simulink model "V2GStronge2_published_controller"  (R2024a)
settings: Solver=odeN  StartTime=0.0  StopTime=36000  FixedStep=10
model workspace (MAT data in the model file):
  Soc = 75
undefined symbols (not defined in the file): Ion, Lithium
libraries: spsMosfetLib x14, spsSeriesRLCBranchLib x14, slpidlib x8, spsBatteryLib x4, spsPWMGeneratorDCDCLib x4, spsCurrentMeasurementLib x3, spsAlphaBetaZerotodq0Lib x2, spsGroundLib x1, spsPWMGenerator2LevelLib x1, eePowerMeasurement x1, spsThreePhaseVIMeasurementLib x1, spsThreePhaseSourceLib x1
(part 2 of 2)

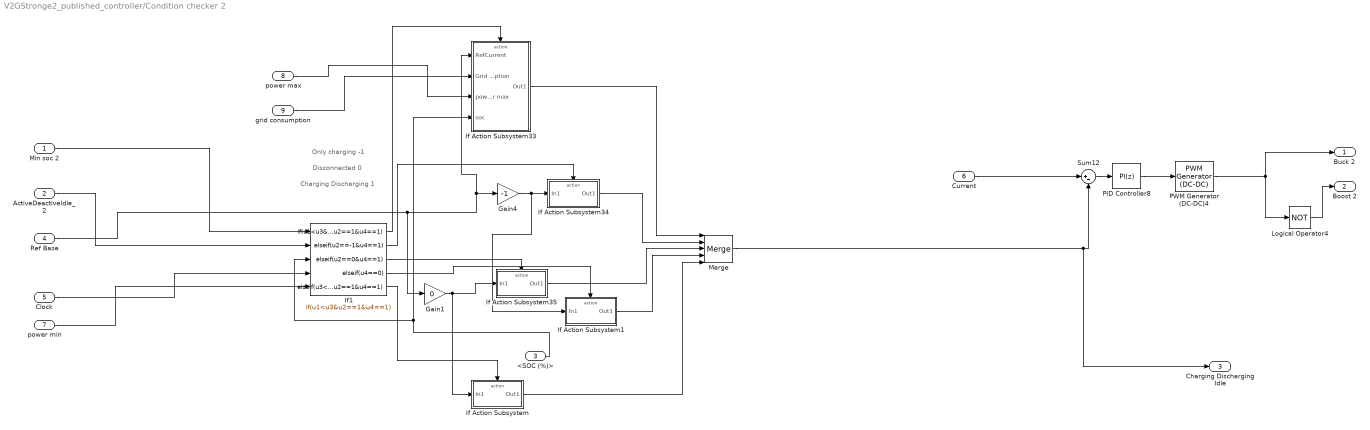
== system V2GStronge2_published_controller/Condition checker 2 ==
  note: Charging Discharging 1
  note: Disconnected 0
  note: Only charging -1
  Min soc 2 : Inport
  ActiveDeactiveIdle_2 : Inport  Port=2
  <SOC (%)> : Inport  Port=3
  Ref Base : Inport  Port=4
  Clock : Inport  Port=5
  Current : Inport  Port=6
  power min : Inport  Port=7
  power max : Inport  Port=8
  grid consumption : Inport  Port=9
  Gain1 : Gain  Gain=0
  Gain4 : Gain  Gain=-1
  If Action Subsystem : Subsystem  TreatAsAtomicUnit=on
  If Action Subsystem1 : Subsystem  TreatAsAtomicUnit=on
  If Action Subsystem33 : Subsystem  TreatAsAtomicUnit=on
  If Action Subsystem34 : Subsystem  TreatAsAtomicUnit=on
  If Action Subsystem35 : Subsystem  TreatAsAtomicUnit=on
  If1 : If  NumInputs=5  IfExpression=u1<u3&u2==1&u4==1  ElseIfExpressions=u2==-1&u4==1,u2==0&u4==1,u4==0,u3<u1&u2==1&u4==1  ShowElse=off
  Logical Operator4 : Logic  Operator=NOT  AllPortsSameDT=off  OutDataTypeStr=boolean
  Merge : Merge  Inputs=5
  PID Controller8 : slpidlib/PID Controller  Controller=PI  Form=Parallel  TimeDomain=Discrete-time  UseExternalTs=off  SampleTime=-1  IntegratorMethod=Forward Euler  FilterMethod=Forward Euler  ControllerParametersSource=internal  P=0.005  I=10  UseKiTs=off  D=0  UseExternalDerivativeSource=off  N=100  UseFilter=on  TunerSelectOption=Transfer Function Based (PID Tuner App)  InitialConditionSource=internal  InitialConditionForIntegrator=0  InitialConditionForFilter=0  DifferentiatorICPrevScaledInput=0  ExternalReset=none  TrackingMode=off  Kt=1  LimitOutput=on  SatLimitsSource=internal  UpperSaturationLimit=0.95  LowerSaturationLimit=0  LinearizeAsGain=on  AntiWindupMode=none  Kb=1  LimitIntegrator=off  UpperIntegratorSaturationLimit=inf  LowerIntegratorSaturationLimit=-inf  POutMin=[]  POutMax=[]  IOutMin=[]  IOutMax=[]  DOutMin=[]  DOutMax=[]  NOutMin=[]  NOutMax=[]  SumOutMin=[]  SumOutMax=[]  SaturationOutMin=[]  SaturationOutMax=[]  PParamMin=[]  PParamMax=[]  IParamMin=[]  IParamMax=[]  DParamMin=[]  DParamMax=[]  NParamMin=[]  NParamMax=[]  KbParamMin=[]  KbParamMax=[]  KtParamMin=[]  KtParamMax=[]  KbOutMin=[]  KbOutMax=[]  KtOutMin=[]  KtOutMax=[]  IntegratorOutMin=[]  IntegratorOutMax=[]  FilterOutMin=[]  FilterOutMax=[]  SumI1OutMin=[]  SumI1OutMax=[]  SumI2OutMin=[]  SumI2OutMax=[]  SumI3OutMin=[]  SumI3OutMax=[]  SumI4OutMin=[]  SumI4OutMax=[]  SumDOutMin=[]  SumDOutMax=[]  DifferentiatorOutMin=[]  DifferentiatorOutMax=[]  FilterDiffOutCoefMin=[]  FilterDiffOutCoefMax=[]  ReciprocalOutMin=[]  ReciprocalOutMax=[]  SumDenOutMin=[]  SumDenOutMax=[]  SumNumOutMin=[]  SumNumOutMax=[]  DivideOutMin=[]  DivideOutMax=[]  UdiffTsProdOutMin=[]  UdiffTsProdOutMax=[]  NTsProdOutMin=[]  NTsProdOutMax=[]  UintegralTsProdOutMin=[]  UintegralTsProdOutMax=[]  UngainTsProdOutMin=[]  UngainTsProdOutMax=[]  ClampingZeroOutDataTypeStr=Inherit: Inherit via back propagation  ClampingZeroOutMin=[]  ClampingZeroOutMax=[]  FilterDenConstantOutDataTypeStr=Inherit: Inherit via back propagation  FilterDenConstantOutMin=[]  FilterDenConstantOutMax=[]  PCopyOutDataTypeStr=Inherit: Inherit via back propagation  PCopyOutMin=[]  PCopyOutMax=[]  NCopyOutDataTypeStr=Inherit: Inherit via back propagation  NCopyOutMin=[]  NCopyOutMax=[]  IntegratorContinuousStateAttributes=''  IntegratorStateMustResolveToSignalObject=off  IntegratorRTWStateStorageClass=Auto  FilterContinuousStateAttributes=''  FilterStateMustResolveToSignalObject=off  FilterRTWStateStorageClass=Auto  ParallelPVariant=InternalParameters  IdealPVariant=Disabled  IVariant=InternalParameters  DVariant=Disabled  IntegratorVariant=Discrete  SatVariant=Enabled  AWVariant=Passthrough  PCopyVariant=Disabled  TRVariant=Disabled  FdbkBlocksVariant=Forward  IdealPFdbkVariant=Disabled  SatFdbkVariant=Disabled  DerivativeFilterVariant=Disabled  NVariant=Disabled  NCopyVariant=Disabled_SignalSpec  FilterICVariant=Disabled  IntegratorICVariant=InternalICs  ExternalResetVariant=Disabled  TRSumVariant=Passthrough  SumFdbkVariant=Disabled  SumVariant=Sum_PI  TsampFilterVariant=InternalTs  TsampNgainVariant=Passthrough  TsampIntegralVariant=Disabled_SignalSpec  ExternalSaturationOutDataTypeStr=Inherit: Same as second input  DerivativeSourceVariant=Disabled
  PWM Generator (DC-DC)4 : spsPWMGeneratorDCDCLib/PWM Generator (DC-DC)  Fsw=60  Ts=0
  Sum12 : Sum  Inputs=|+-
  Buck 2 : Outport
  Boost 2 : Outport  Port=2
  Charging Discharging Idle : Outport  Port=3
  wires:
  Current/1 -> Sum12/1
  Sum12/1 -> PID Controller8/1
  If1/3 -> If Action Subsystem35/Action
  PID Controller8/1 -> PWM Generator (DC-DC)4/1
  If1/1 -> If Action Subsystem33/Action
  grid consumption/1 -> If Action Subsystem33/2(Grid Consumption)
  If Action Subsystem35/1(Out1) -> Merge/3
  Min soc 2/1 -> If1/1
  Logical Operator4/1 -> Boost 2/1
  Ref Base/1 -> If Action Subsystem33/1(RefCurrent), Gain4/1, Gain1/1
  If Action Subsystem33/1(Out1) -> Merge/1
  Gain4/1 -> If Action Subsystem1/1(In1), If Action Subsystem34/1(In1)
  ActiveDeactiveIdle_2/1 -> If1/2
  PWM Generator (DC-DC)4/1 -> Buck 2/1, Logical Operator4/1
  If Action Subsystem34/1(Out1) -> Merge/2
  If1/2 -> If Action Subsystem34/Action
  power max/1 -> If Action Subsystem33/3(power max)
  <SOC (%)>/1 -> If Action Subsystem33/4(soc), If1/3
  Clock/1 -> If1/4
  If Action Subsystem1/1(Out1) -> Merge/4
  If1/4 -> If Action Subsystem1/Action
  power min/1 -> If1/5
  Merge/1 -> Charging Discharging Idle/1, Sum12/2
  Gain1/1 -> If Action Subsystem/1(In1), If Action Subsystem35/1(In1)
  If1/5 -> If Action Subsystem/Action
  If Action Subsystem/1(Out1) -> Merge/5

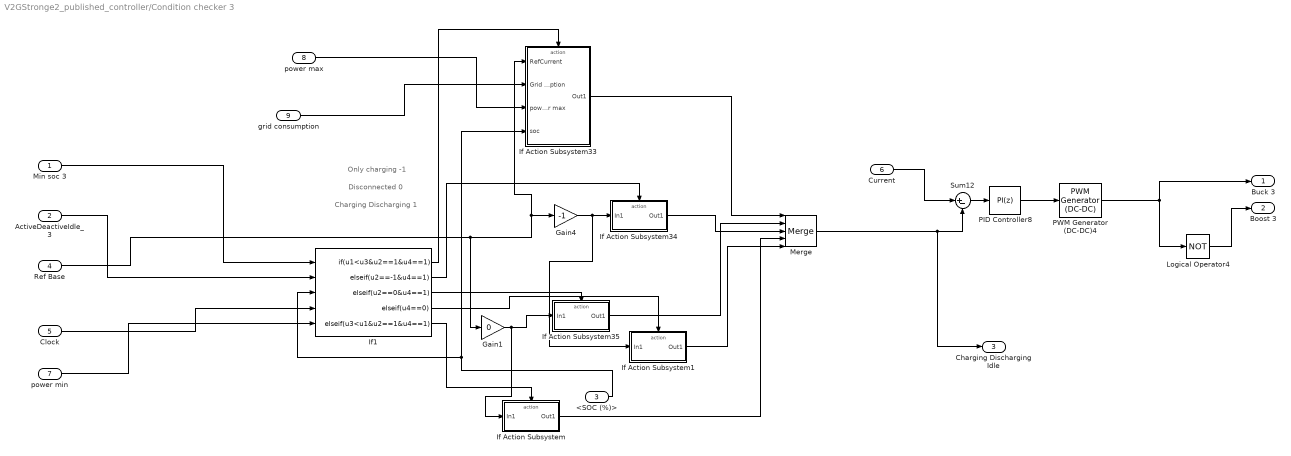
== system V2GStronge2_published_controller/Condition checker 3 ==
  note: Charging Discharging 1
  note: Disconnected 0
  note: Only charging -1
  Min soc 3 : Inport
  ActiveDeactiveIdle_3 : Inport  Port=2
  <SOC (%)> : Inport  Port=3
  Ref Base : Inport  Port=4
  Clock : Inport  Port=5
  Current : Inport  Port=6
  power min : Inport  Port=7
  power max : Inport  Port=8
  grid consumption : Inport  Port=9
  Gain1 : Gain  Gain=0
  Gain4 : Gain  Gain=-1
  If Action Subsystem : Subsystem  TreatAsAtomicUnit=on
  If Action Subsystem1 : Subsystem  TreatAsAtomicUnit=on
  If Action Subsystem33 : Subsystem  TreatAsAtomicUnit=on
  If Action Subsystem34 : Subsystem  TreatAsAtomicUnit=on
  If Action Subsystem35 : Subsystem  TreatAsAtomicUnit=on
  If1 : If  NumInputs=5  IfExpression=u1<u3&u2==1&u4==1  ElseIfExpressions=u2==-1&u4==1,u2==0&u4==1,u4==0,u3<u1&u2==1&u4==1  ShowElse=off
  Logical Operator4 : Logic  Operator=NOT  AllPortsSameDT=off  OutDataTypeStr=boolean
  Merge : Merge  Inputs=5
  PID Controller8 : slpidlib/PID Controller  Controller=PI  Form=Parallel  TimeDomain=Discrete-time  UseExternalTs=off  SampleTime=-1  IntegratorMethod=Forward Euler  FilterMethod=Forward Euler  ControllerParametersSource=internal  P=0.005  I=10  UseKiTs=off  D=0  UseExternalDerivativeSource=off  N=100  UseFilter=on  TunerSelectOption=Transfer Function Based (PID Tuner App)  InitialConditionSource=internal  InitialConditionForIntegrator=0  InitialConditionForFilter=0  DifferentiatorICPrevScaledInput=0  ExternalReset=none  TrackingMode=off  Kt=1  LimitOutput=on  SatLimitsSource=internal  UpperSaturationLimit=0.95  LowerSaturationLimit=0  LinearizeAsGain=on  AntiWindupMode=none  Kb=1  LimitIntegrator=off  UpperIntegratorSaturationLimit=inf  LowerIntegratorSaturationLimit=-inf  POutMin=[]  POutMax=[]  IOutMin=[]  IOutMax=[]  DOutMin=[]  DOutMax=[]  NOutMin=[]  NOutMax=[]  SumOutMin=[]  SumOutMax=[]  SaturationOutMin=[]  SaturationOutMax=[]  PParamMin=[]  PParamMax=[]  IParamMin=[]  IParamMax=[]  DParamMin=[]  DParamMax=[]  NParamMin=[]  NParamMax=[]  KbParamMin=[]  KbParamMax=[]  KtParamMin=[]  KtParamMax=[]  KbOutMin=[]  KbOutMax=[]  KtOutMin=[]  KtOutMax=[]  IntegratorOutMin=[]  IntegratorOutMax=[]  FilterOutMin=[]  FilterOutMax=[]  SumI1OutMin=[]  SumI1OutMax=[]  SumI2OutMin=[]  SumI2OutMax=[]  SumI3OutMin=[]  SumI3OutMax=[]  SumI4OutMin=[]  SumI4OutMax=[]  SumDOutMin=[]  SumDOutMax=[]  DifferentiatorOutMin=[]  DifferentiatorOutMax=[]  FilterDiffOutCoefMin=[]  FilterDiffOutCoefMax=[]  ReciprocalOutMin=[]  ReciprocalOutMax=[]  SumDenOutMin=[]  SumDenOutMax=[]  SumNumOutMin=[]  SumNumOutMax=[]  DivideOutMin=[]  DivideOutMax=[]  UdiffTsProdOutMin=[]  UdiffTsProdOutMax=[]  NTsProdOutMin=[]  NTsProdOutMax=[]  UintegralTsProdOutMin=[]  UintegralTsProdOutMax=[]  UngainTsProdOutMin=[]  UngainTsProdOutMax=[]  ClampingZeroOutDataTypeStr=Inherit: Inherit via back propagation  ClampingZeroOutMin=[]  ClampingZeroOutMax=[]  FilterDenConstantOutDataTypeStr=Inherit: Inherit via back propagation  FilterDenConstantOutMin=[]  FilterDenConstantOutMax=[]  PCopyOutDataTypeStr=Inherit: Inherit via back propagation  PCopyOutMin=[]  PCopyOutMax=[]  NCopyOutDataTypeStr=Inherit: Inherit via back propagation  NCopyOutMin=[]  NCopyOutMax=[]  IntegratorContinuousStateAttributes=''  IntegratorStateMustResolveToSignalObject=off  IntegratorRTWStateStorageClass=Auto  FilterContinuousStateAttributes=''  FilterStateMustResolveToSignalObject=off  FilterRTWStateStorageClass=Auto  ParallelPVariant=InternalParameters  IdealPVariant=Disabled  IVariant=InternalParameters  DVariant=Disabled  IntegratorVariant=Discrete  SatVariant=Enabled  AWVariant=Passthrough  PCopyVariant=Disabled  TRVariant=Disabled  FdbkBlocksVariant=Forward  IdealPFdbkVariant=Disabled  SatFdbkVariant=Disabled  DerivativeFilterVariant=Disabled  NVariant=Disabled  NCopyVariant=Disabled_SignalSpec  FilterICVariant=Disabled  IntegratorICVariant=InternalICs  ExternalResetVariant=Disabled  TRSumVariant=Passthrough  SumFdbkVariant=Disabled  SumVariant=Sum_PI  TsampFilterVariant=InternalTs  TsampNgainVariant=Passthrough  TsampIntegralVariant=Disabled_SignalSpec  ExternalSaturationOutDataTypeStr=Inherit: Same as second input  DerivativeSourceVariant=Disabled
  PWM Generator (DC-DC)4 : spsPWMGeneratorDCDCLib/PWM Generator (DC-DC)  Fsw=60  Ts=0
  Sum12 : Sum  Inputs=|+-
  Buck 3 : Outport
  Boost 3 : Outport  Port=2
  Charging Discharging Idle : Outport  Port=3
  wires:
  Current/1 -> Sum12/1
  Sum12/1 -> PID Controller8/1
  If1/3 -> If Action Subsystem35/Action
  PID Controller8/1 -> PWM Generator (DC-DC)4/1
  If1/1 -> If Action Subsystem33/Action
  grid consumption/1 -> If Action Subsystem33/2(Grid Consumption)
  If Action Subsystem35/1(Out1) -> Merge/2
  Min soc 3/1 -> If1/1
  Logical Operator4/1 -> Boost 3/1
  Ref Base/1 -> Gain1/1, If Action Subsystem33/1(RefCurrent), Gain4/1
  If Action Subsystem33/1(Out1) -> Merge/1
  Gain4/1 -> If Action Subsystem1/1(In1), If Action Subsystem34/1(In1)
  ActiveDeactiveIdle_3/1 -> If1/2
  PWM Generator (DC-DC)4/1 -> Buck 3/1, Logical Operator4/1
  Gain1/1 -> If Action Subsystem/1(In1), If Action Subsystem35/1(In1)
  If Action Subsystem34/1(Out1) -> Merge/3
  If1/2 -> If Action Subsystem34/Action
  power max/1 -> If Action Subsystem33/3(power max)
  <SOC (%)>/1 -> If Action Subsystem33/4(soc), If1/3
  Clock/1 -> If1/4
  If Action Subsystem1/1(Out1) -> Merge/5
  If1/4 -> If Action Subsystem1/Action
  power min/1 -> If1/5
  Merge/1 -> Charging Discharging Idle/1, Sum12/2
  If1/5 -> If Action Subsystem/Action
  If Action Subsystem/1(Out1) -> Merge/4

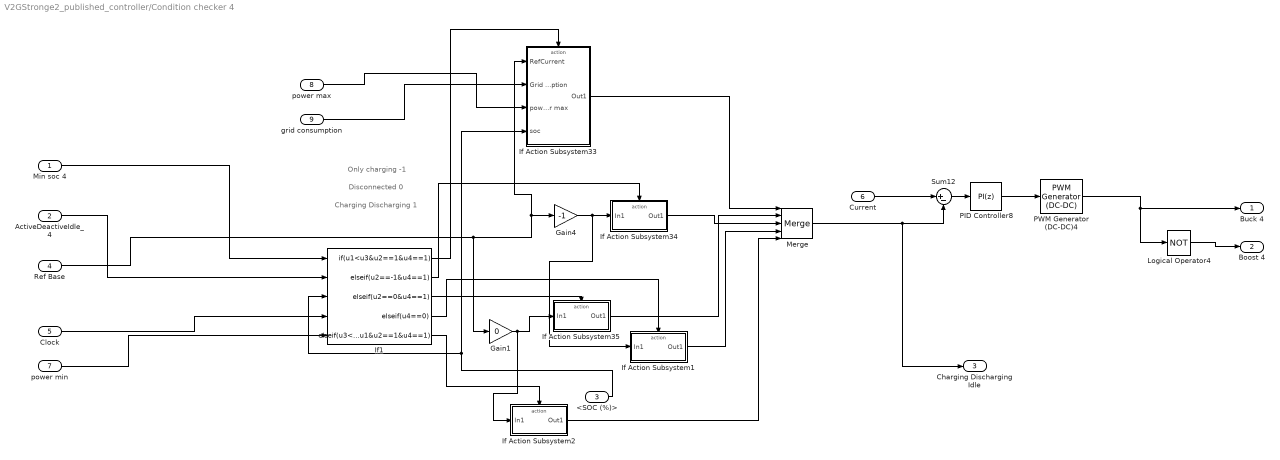
== system V2GStronge2_published_controller/Condition checker 4 ==
  note: Charging Discharging 1
  note: Disconnected 0
  note: Only charging -1
  Min soc 4 : Inport
  ActiveDeactiveIdle_4 : Inport  Port=2
  <SOC (%)> : Inport  Port=3
  Ref Base : Inport  Port=4
  Clock : Inport  Port=5
  Current : Inport  Port=6
  power min : Inport  Port=7
  power max : Inport  Port=8
  grid consumption : Inport  Port=9
  Gain1 : Gain  Gain=0
  Gain4 : Gain  Gain=-1
  If Action Subsystem1 : Subsystem  TreatAsAtomicUnit=on
  If Action Subsystem2 : Subsystem  TreatAsAtomicUnit=on
  If Action Subsystem33 : Subsystem  TreatAsAtomicUnit=on
  If Action Subsystem34 : Subsystem  TreatAsAtomicUnit=on
  If Action Subsystem35 : Subsystem  TreatAsAtomicUnit=on
  If1 : If  NumInputs=5  IfExpression=u1<u3&u2==1&u4==1  ElseIfExpressions=u2==-1&u4==1,u2==0&u4==1,u4==0,u3<u1&u2==1&u4==1  ShowElse=off
  Logical Operator4 : Logic  Operator=NOT  AllPortsSameDT=off  OutDataTypeStr=boolean
  Merge : Merge  Inputs=5
  PID Controller8 : slpidlib/PID Controller  Controller=PI  Form=Parallel  TimeDomain=Discrete-time  UseExternalTs=off  SampleTime=-1  IntegratorMethod=Forward Euler  FilterMethod=Forward Euler  ControllerParametersSource=internal  P=0.005  I=10  UseKiTs=off  D=0  UseExternalDerivativeSource=off  N=100  UseFilter=on  TunerSelectOption=Transfer Function Based (PID Tuner App)  InitialConditionSource=internal  InitialConditionForIntegrator=0  InitialConditionForFilter=0  DifferentiatorICPrevScaledInput=0  ExternalReset=none  TrackingMode=off  Kt=1  LimitOutput=on  SatLimitsSource=internal  UpperSaturationLimit=0.95  LowerSaturationLimit=0  LinearizeAsGain=on  AntiWindupMode=none  Kb=1  LimitIntegrator=off  UpperIntegratorSaturationLimit=inf  LowerIntegratorSaturationLimit=-inf  POutMin=[]  POutMax=[]  IOutMin=[]  IOutMax=[]  DOutMin=[]  DOutMax=[]  NOutMin=[]  NOutMax=[]  SumOutMin=[]  SumOutMax=[]  SaturationOutMin=[]  SaturationOutMax=[]  PParamMin=[]  PParamMax=[]  IParamMin=[]  IParamMax=[]  DParamMin=[]  DParamMax=[]  NParamMin=[]  NParamMax=[]  KbParamMin=[]  KbParamMax=[]  KtParamMin=[]  KtParamMax=[]  KbOutMin=[]  KbOutMax=[]  KtOutMin=[]  KtOutMax=[]  IntegratorOutMin=[]  IntegratorOutMax=[]  FilterOutMin=[]  FilterOutMax=[]  SumI1OutMin=[]  SumI1OutMax=[]  SumI2OutMin=[]  SumI2OutMax=[]  SumI3OutMin=[]  SumI3OutMax=[]  SumI4OutMin=[]  SumI4OutMax=[]  SumDOutMin=[]  SumDOutMax=[]  DifferentiatorOutMin=[]  DifferentiatorOutMax=[]  FilterDiffOutCoefMin=[]  FilterDiffOutCoefMax=[]  ReciprocalOutMin=[]  ReciprocalOutMax=[]  SumDenOutMin=[]  SumDenOutMax=[]  SumNumOutMin=[]  SumNumOutMax=[]  DivideOutMin=[]  DivideOutMax=[]  UdiffTsProdOutMin=[]  UdiffTsProdOutMax=[]  NTsProdOutMin=[]  NTsProdOutMax=[]  UintegralTsProdOutMin=[]  UintegralTsProdOutMax=[]  UngainTsProdOutMin=[]  UngainTsProdOutMax=[]  ClampingZeroOutDataTypeStr=Inherit: Inherit via back propagation  ClampingZeroOutMin=[]  ClampingZeroOutMax=[]  FilterDenConstantOutDataTypeStr=Inherit: Inherit via back propagation  FilterDenConstantOutMin=[]  FilterDenConstantOutMax=[]  PCopyOutDataTypeStr=Inherit: Inherit via back propagation  PCopyOutMin=[]  PCopyOutMax=[]  NCopyOutDataTypeStr=Inherit: Inherit via back propagation  NCopyOutMin=[]  NCopyOutMax=[]  IntegratorContinuousStateAttributes=''  IntegratorStateMustResolveToSignalObject=off  IntegratorRTWStateStorageClass=Auto  FilterContinuousStateAttributes=''  FilterStateMustResolveToSignalObject=off  FilterRTWStateStorageClass=Auto  ParallelPVariant=InternalParameters  IdealPVariant=Disabled  IVariant=InternalParameters  DVariant=Disabled  IntegratorVariant=Discrete  SatVariant=Enabled  AWVariant=Passthrough  PCopyVariant=Disabled  TRVariant=Disabled  FdbkBlocksVariant=Forward  IdealPFdbkVariant=Disabled  SatFdbkVariant=Disabled  DerivativeFilterVariant=Disabled  NVariant=Disabled  NCopyVariant=Disabled_SignalSpec  FilterICVariant=Disabled  IntegratorICVariant=InternalICs  ExternalResetVariant=Disabled  TRSumVariant=Passthrough  SumFdbkVariant=Disabled  SumVariant=Sum_PI  TsampFilterVariant=InternalTs  TsampNgainVariant=Passthrough  TsampIntegralVariant=Disabled_SignalSpec  ExternalSaturationOutDataTypeStr=Inherit: Same as second input  DerivativeSourceVariant=Disabled
  PWM Generator (DC-DC)4 : spsPWMGeneratorDCDCLib/PWM Generator (DC-DC)  Fsw=60  Ts=0
  Sum12 : Sum  Inputs=|+-
  Buck 4 : Outport
  Boost 4 : Outport  Port=2
  Charging Discharging Idle : Outport  Port=3
  wires:
  Current/1 -> Sum12/1
  Sum12/1 -> PID Controller8/1
  If1/3 -> If Action Subsystem35/Action
  PID Controller8/1 -> PWM Generator (DC-DC)4/1
  If1/1 -> If Action Subsystem33/Action
  grid consumption/1 -> If Action Subsystem33/2(Grid Consumption)
  If Action Subsystem35/1(Out1) -> Merge/2
  Min soc 4/1 -> If1/1
  Ref Base/1 -> Gain1/1, If Action Subsystem33/1(RefCurrent), Gain4/1
  If Action Subsystem33/1(Out1) -> Merge/1
  Gain4/1 -> If Action Subsystem1/1(In1), If Action Subsystem34/1(In1)
  ActiveDeactiveIdle_4/1 -> If1/2
  PWM Generator (DC-DC)4/1 -> Buck 4/1, Logical Operator4/1
  Gain1/1 -> If Action Subsystem2/1(In1), If Action Subsystem35/1(In1)
  If Action Subsystem34/1(Out1) -> Merge/3
  If1/2 -> If Action Subsystem34/Action
  power max/1 -> If Action Subsystem33/3(power max)
  <SOC (%)>/1 -> If Action Subsystem33/4(soc), If1/3
  Clock/1 -> If1/4
  If Action Subsystem1/1(Out1) -> Merge/4
  If1/4 -> If Action Subsystem1/Action
  Logical Operator4/1 -> Boost 4/1
  power min/1 -> If1/5
  Merge/1 -> Charging Discharging Idle/1, Sum12/2
  If1/5 -> If Action Subsystem2/Action
  If Action Subsystem2/1(Out1) -> Merge/5

== system V2GStronge2_published_controller/Charge//Discharge//Ideal Detection/If Action Subsystem ==
  In1 : Inport
  Action Port : ActionPort  ActionPortLabel=if(u1 > 0)
  Out1 : Outport
  wires:
  In1/1 -> Out1/1

== system V2GStronge2_published_controller/Charge//Discharge//Ideal Detection/If Action Subsystem1 ==
  In1 : Inport
  Action Port : ActionPort  ActionPortLabel=elseif( u1==0)
  Out1 : Outport
  wires:
  In1/1 -> Out1/1

== system V2GStronge2_published_controller/Charge//Discharge//Ideal Detection/If Action Subsystem2 ==
  In1 : Inport
  Action Port : ActionPort  ActionPortLabel=elseif(u1<0)
  Out1 : Outport
  wires:
  In1/1 -> Out1/1

== system V2GStronge2_published_controller/Charge//Discharge//Ideal Detection1/If Action Subsystem ==
  In1 : Inport
  Action Port : ActionPort  ActionPortLabel=if(u1 > 0)
  Out1 : Outport
  wires:
  In1/1 -> Out1/1

== system V2GStronge2_published_controller/Charge//Discharge//Ideal Detection1/If Action Subsystem1 ==
  In1 : Inport
  Action Port : ActionPort  ActionPortLabel=elseif( u1==0)
  Out1 : Outport
  wires:
  In1/1 -> Out1/1

== system V2GStronge2_published_controller/Charge//Discharge//Ideal Detection1/If Action Subsystem2 ==
  In1 : Inport
  Action Port : ActionPort  ActionPortLabel=elseif(u1<0)
  Out1 : Outport
  wires:
  In1/1 -> Out1/1

== system V2GStronge2_published_controller/Charge//Discharge//Ideal Detection2/If Action Subsystem ==
  In1 : Inport
  Action Port : ActionPort  ActionPortLabel=if(u1 > 0)
  Out1 : Outport
  wires:
  In1/1 -> Out1/1

== system V2GStronge2_published_controller/Charge//Discharge//Ideal Detection2/If Action Subsystem1 ==
  In1 : Inport
  Action Port : ActionPort  ActionPortLabel=elseif( u1==0)
  Out1 : Outport
  wires:
  In1/1 -> Out1/1

== system V2GStronge2_published_controller/Charge//Discharge//Ideal Detection2/If Action Subsystem2 ==
  In1 : Inport
  Action Port : ActionPort  ActionPortLabel=elseif(u1<0)
  Out1 : Outport
  wires:
  In1/1 -> Out1/1

== system V2GStronge2_published_controller/Charge//Discharge//Ideal Detection3/If Action Subsystem ==
  In1 : Inport
  Action Port : ActionPort  ActionPortLabel=if(u1 > 0)
  Out1 : Outport
  wires:
  In1/1 -> Out1/1

== system V2GStronge2_published_controller/Charge//Discharge//Ideal Detection3/If Action Subsystem1 ==
  In1 : Inport
  Action Port : ActionPort  ActionPortLabel=elseif( u1==0)
  Out1 : Outport
  wires:
  In1/1 -> Out1/1

== system V2GStronge2_published_controller/Charge//Discharge//Ideal Detection3/If Action Subsystem2 ==
  In1 : Inport
  Action Port : ActionPort  ActionPortLabel=elseif(u1<0)
  Out1 : Outport
  wires:
  In1/1 -> Out1/1

== system V2GStronge2_published_controller/Condition checker 1/If Action Subsystem ==
  In1 : Inport
  Action Port : ActionPort  ActionPortLabel=elseif(u3<u1&u2==1&u4==1)
  Out1 : Outport
  wires:
  In1/1 -> Out1/1

== system V2GStronge2_published_controller/Condition checker 1/If Action Subsystem1 ==
  In1 : Inport
  Action Port : ActionPort  PropagateVarSize=During execution  ActionPortLabel=elseif(u4==0)
  Out1 : Outport
  wires:
  In1/1 -> Out1/1

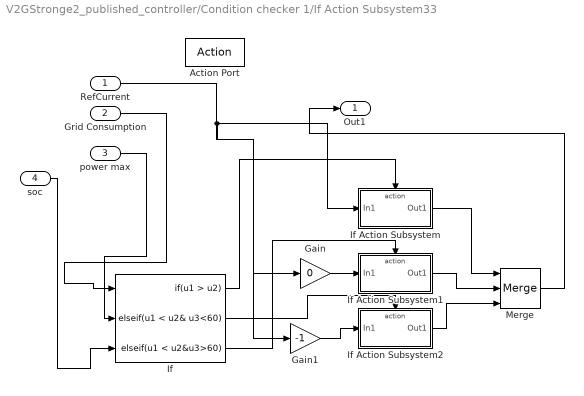
== system V2GStronge2_published_controller/Condition checker 1/If Action Subsystem33 ==
  RefCurrent : Inport
  Grid Consumption : Inport  Port=2
  power max : Inport  Port=3
  soc : Inport  Port=4
  Action Port : ActionPort  PropagateVarSize=During execution  ActionPortLabel=if(u1<u3&u2==1&u4==1)
  Gain : Gain  Gain=0
  Gain1 : Gain  Gain=-1
  If : If  NumInputs=3  IfExpression=u1 > u2  ElseIfExpressions=u1 < u2& u3<60, u1 < u2&u3>60  ShowElse=off
  If Action Subsystem : Subsystem  TreatAsAtomicUnit=on
  If Action Subsystem1 : Subsystem  TreatAsAtomicUnit=on
  If Action Subsystem2 : Subsystem  TreatAsAtomicUnit=on
  Merge : Merge  Inputs=3
  Out1 : Outport
  wires:
  RefCurrent/1 -> Gain/1, Gain1/1, If Action Subsystem/1(In1)
  Grid Consumption/1 -> If/1
  power max/1 -> If/2
  If/1 -> If Action Subsystem/Action
  soc/1 -> If/3
  If Action Subsystem/1(Out1) -> Merge/1
  If/2 -> If Action Subsystem2/Action
  Gain/1 -> If Action Subsystem1/1(In1)
  If Action Subsystem1/1(Out1) -> Merge/2
  Merge/1 -> Out1/1
  If Action Subsystem2/1(Out1) -> Merge/3
  If/3 -> If Action Subsystem1/Action
  Gain1/1 -> If Action Subsystem2/1(In1)

== system V2GStronge2_published_controller/Condition checker 1/If Action Subsystem34 ==
  In1 : Inport
  Action Port : ActionPort  PropagateVarSize=During execution  ActionPortLabel=elseif(u2==-1&u4==1)
  Out1 : Outport
  wires:
  In1/1 -> Out1/1

== system V2GStronge2_published_controller/Condition checker 1/If Action Subsystem35 ==
  In1 : Inport
  Action Port : ActionPort  PropagateVarSize=During execution  ActionPortLabel=elseif(u2==0&u4==1)
  Out1 : Outport
  wires:
  In1/1 -> Out1/1

== system V2GStronge2_published_controller/Condition checker 2/If Action Subsystem ==
  In1 : Inport
  Action Port : ActionPort  ActionPortLabel=elseif(u3<u1&u2==1&u4==1)
  Out1 : Outport
  wires:
  In1/1 -> Out1/1

== system V2GStronge2_published_controller/Condition checker 2/If Action Subsystem1 ==
  In1 : Inport
  Action Port : ActionPort  ActionPortLabel=elseif(u4==0)
  Out1 : Outport
  wires:
  In1/1 -> Out1/1

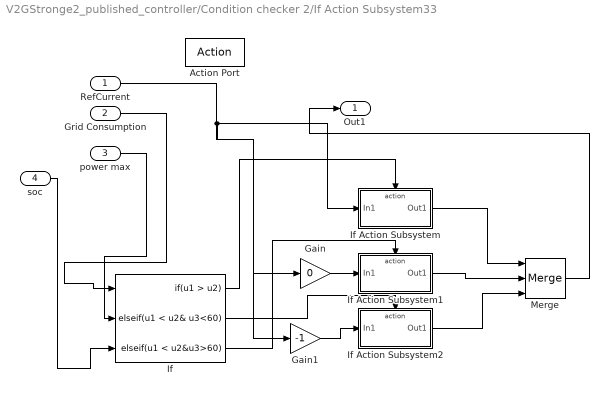
== system V2GStronge2_published_controller/Condition checker 2/If Action Subsystem33 ==
  RefCurrent : Inport
  Grid Consumption : Inport  Port=2
  power max : Inport  Port=3
  soc : Inport  Port=4
  Action Port : ActionPort  ActionPortLabel=if(u1<u3&u2==1&u4==1)
  Gain : Gain  Gain=0
  Gain1 : Gain  Gain=-1
  If : If  NumInputs=3  IfExpression=u1 > u2  ElseIfExpressions=u1 < u2& u3<60, u1 < u2&u3>60  ShowElse=off
  If Action Subsystem : Subsystem  TreatAsAtomicUnit=on
  If Action Subsystem1 : Subsystem  TreatAsAtomicUnit=on
  If Action Subsystem2 : Subsystem  TreatAsAtomicUnit=on
  Merge : Merge  Inputs=3
  Out1 : Outport
  wires:
  RefCurrent/1 -> Gain/1, Gain1/1, If Action Subsystem/1(In1)
  Grid Consumption/1 -> If/1
  power max/1 -> If/2
  If/1 -> If Action Subsystem/Action
  soc/1 -> If/3
  If Action Subsystem/1(Out1) -> Merge/1
  If/2 -> If Action Subsystem2/Action
  Gain/1 -> If Action Subsystem1/1(In1)
  If Action Subsystem1/1(Out1) -> Merge/2
  Merge/1 -> Out1/1
  If Action Subsystem2/1(Out1) -> Merge/3
  If/3 -> If Action Subsystem1/Action
  Gain1/1 -> If Action Subsystem2/1(In1)

== system V2GStronge2_published_controller/Condition checker 2/If Action Subsystem34 ==
  In1 : Inport
  Action Port : ActionPort  ActionPortLabel=elseif(u2==-1&u4==1)
  Out1 : Outport
  wires:
  In1/1 -> Out1/1

== system V2GStronge2_published_controller/Condition checker 2/If Action Subsystem35 ==
  In1 : Inport
  Action Port : ActionPort  ActionPortLabel=elseif(u2==0&u4==1)
  Out1 : Outport
  wires:
  In1/1 -> Out1/1

== system V2GStronge2_published_controller/Condition checker 3/If Action Subsystem ==
  In1 : Inport
  Action Port : ActionPort  ActionPortLabel=elseif(u3<u1&u2==1&u4==1)
  Out1 : Outport
  wires:
  In1/1 -> Out1/1

== system V2GStronge2_published_controller/Condition checker 3/If Action Subsystem1 ==
  In1 : Inport
  Action Port : ActionPort  ActionPortLabel=elseif(u4==0)
  Out1 : Outport
  wires:
  In1/1 -> Out1/1

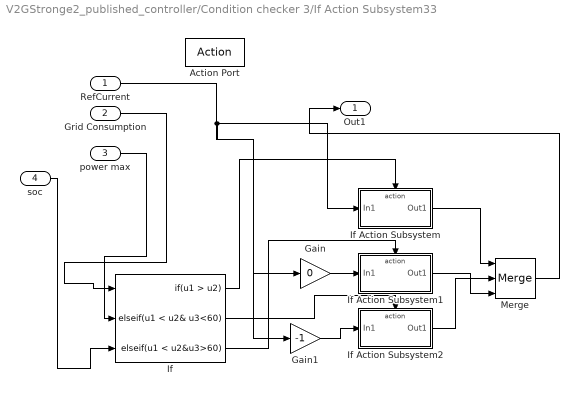
== system V2GStronge2_published_controller/Condition checker 3/If Action Subsystem33 ==
  RefCurrent : Inport
  Grid Consumption : Inport  Port=2
  power max : Inport  Port=3
  soc : Inport  Port=4
  Action Port : ActionPort  ActionPortLabel=if(u1<u3&u2==1&u4==1)
  Gain : Gain  Gain=0
  Gain1 : Gain  Gain=-1
  If : If  NumInputs=3  IfExpression=u1 > u2  ElseIfExpressions=u1 < u2& u3<60, u1 < u2&u3>60  ShowElse=off
  If Action Subsystem : Subsystem  TreatAsAtomicUnit=on
  If Action Subsystem1 : Subsystem  TreatAsAtomicUnit=on
  If Action Subsystem2 : Subsystem  TreatAsAtomicUnit=on
  Merge : Merge  Inputs=3
  Out1 : Outport
  wires:
  RefCurrent/1 -> Gain/1, Gain1/1, If Action Subsystem/1(In1)
  Grid Consumption/1 -> If/1
  power max/1 -> If/2
  If/1 -> If Action Subsystem/Action
  soc/1 -> If/3
  If Action Subsystem/1(Out1) -> Merge/1
  If/2 -> If Action Subsystem2/Action
  Gain/1 -> If Action Subsystem1/1(In1)
  If Action Subsystem1/1(Out1) -> Merge/3
  Merge/1 -> Out1/1
  If Action Subsystem2/1(Out1) -> Merge/2
  If/3 -> If Action Subsystem1/Action
  Gain1/1 -> If Action Subsystem2/1(In1)

== system V2GStronge2_published_controller/Condition checker 3/If Action Subsystem34 ==
  In1 : Inport
  Action Port : ActionPort  ActionPortLabel=elseif(u2==-1&u4==1)
  Out1 : Outport
  wires:
  In1/1 -> Out1/1

== system V2GStronge2_published_controller/Condition checker 3/If Action Subsystem35 ==
  In1 : Inport
  Action Port : ActionPort  ActionPortLabel=elseif(u2==0&u4==1)
  Out1 : Outport
  wires:
  In1/1 -> Out1/1

== system V2GStronge2_published_controller/Condition checker 4/If Action Subsystem1 ==
  In1 : Inport
  Action Port : ActionPort  ActionPortLabel=elseif(u4==0)
  Out1 : Outport
  wires:
  In1/1 -> Out1/1

== system V2GStronge2_published_controller/Condition checker 4/If Action Subsystem2 ==
  In1 : Inport
  Action Port : ActionPort  ActionPortLabel=elseif(u3<u1&u2==1&u4==1)
  Out1 : Outport
  wires:
  In1/1 -> Out1/1

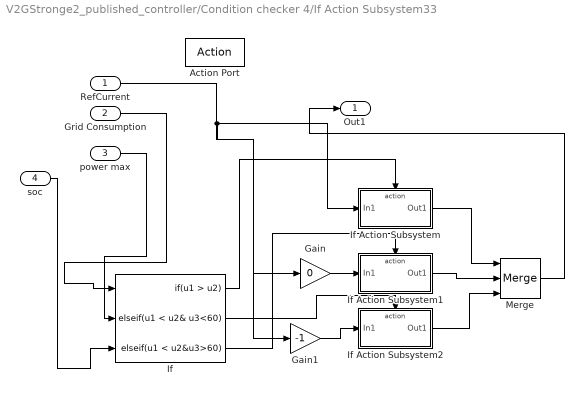
== system V2GStronge2_published_controller/Condition checker 4/If Action Subsystem33 ==
  RefCurrent : Inport
  Grid Consumption : Inport  Port=2
  power max : Inport  Port=3
  soc : Inport  Port=4
  Action Port : ActionPort  ActionPortLabel=if(u1<u3&u2==1&u4==1)
  Gain : Gain  Gain=0
  Gain1 : Gain  Gain=-1
  If : If  NumInputs=3  IfExpression=u1 > u2  ElseIfExpressions=u1 < u2& u3<60, u1 < u2&u3>60  ShowElse=off
  If Action Subsystem : Subsystem  TreatAsAtomicUnit=on
  If Action Subsystem1 : Subsystem  TreatAsAtomicUnit=on
  If Action Subsystem2 : Subsystem  TreatAsAtomicUnit=on
  Merge : Merge  Inputs=3
  Out1 : Outport
  wires:
  RefCurrent/1 -> Gain/1, Gain1/1, If Action Subsystem/1(In1)
  Grid Consumption/1 -> If/1
  power max/1 -> If/2
  If/1 -> If Action Subsystem/Action
  soc/1 -> If/3
  If Action Subsystem/1(Out1) -> Merge/1
  If/2 -> If Action Subsystem2/Action
  Gain/1 -> If Action Subsystem1/1(In1)
  If Action Subsystem1/1(Out1) -> Merge/2
  Merge/1 -> Out1/1
  If Action Subsystem2/1(Out1) -> Merge/3
  If/3 -> If Action Subsystem1/Action
  Gain1/1 -> If Action Subsystem2/1(In1)

== system V2GStronge2_published_controller/Condition checker 4/If Action Subsystem34 ==
  In1 : Inport
  Action Port : ActionPort  ActionPortLabel=elseif(u2==-1&u4==1)
  Out1 : Outport
  wires:
  In1/1 -> Out1/1

== system V2GStronge2_published_controller/Condition checker 4/If Action Subsystem35 ==
  In1 : Inport
  Action Port : ActionPort  ActionPortLabel=elseif(u2==0&u4==1)
  Out1 : Outport
  wires:
  In1/1 -> Out1/1

== system V2GStronge2_published_controller/Condition checker 1/If Action Subsystem33/If Action Subsystem ==
  In1 : Inport
  Action Port : ActionPort  InitializeStates=reset  ActionPortLabel=if(u1 > u2)
  Out1 : Outport
  wires:
  In1/1 -> Out1/1

== system V2GStronge2_published_controller/Condition checker 1/If Action Subsystem33/If Action Subsystem1 ==
  In1 : Inport
  Action Port : ActionPort  InitializeStates=reset  PropagateVarSize=During execution  ActionPortLabel=elseif( u1 < u2&u3>60)
  Out1 : Outport
  wires:
  In1/1 -> Out1/1

== system V2GStronge2_published_controller/Condition checker 1/If Action Subsystem33/If Action Subsystem2 ==
  In1 : Inport
  Action Port : ActionPort  InitializeStates=reset  PropagateVarSize=During execution  ActionPortLabel=elseif(u1 < u2& u3<60)
  Out1 : Outport
  wires:
  In1/1 -> Out1/1

== system V2GStronge2_published_controller/Condition checker 2/If Action Subsystem33/If Action Subsystem ==
  In1 : Inport
  Action Port : ActionPort  ActionPortLabel=if(u1 > u2)
  Out1 : Outport
  wires:
  In1/1 -> Out1/1

== system V2GStronge2_published_controller/Condition checker 2/If Action Subsystem33/If Action Subsystem1 ==
  In1 : Inport
  Action Port : ActionPort  ActionPortLabel=elseif( u1 < u2&u3>60)
  Out1 : Outport
  wires:
  In1/1 -> Out1/1

== system V2GStronge2_published_controller/Condition checker 2/If Action Subsystem33/If Action Subsystem2 ==
  In1 : Inport
  Action Port : ActionPort  ActionPortLabel=elseif(u1 < u2& u3<60)
  Out1 : Outport
  wires:
  In1/1 -> Out1/1

== system V2GStronge2_published_controller/Condition checker 3/If Action Subsystem33/If Action Subsystem ==
  In1 : Inport
  Action Port : ActionPort  ActionPortLabel=if(u1 > u2)
  Out1 : Outport
  wires:
  In1/1 -> Out1/1

== system V2GStronge2_published_controller/Condition checker 3/If Action Subsystem33/If Action Subsystem1 ==
  In1 : Inport
  Action Port : ActionPort  ActionPortLabel=elseif( u1 < u2&u3>60)
  Out1 : Outport
  wires:
  In1/1 -> Out1/1

== system V2GStronge2_published_controller/Condition checker 3/If Action Subsystem33/If Action Subsystem2 ==
  In1 : Inport
  Action Port : ActionPort  ActionPortLabel=elseif(u1 < u2& u3<60)
  Out1 : Outport
  wires:
  In1/1 -> Out1/1

== system V2GStronge2_published_controller/Condition checker 4/If Action Subsystem33/If Action Subsystem ==
  In1 : Inport
  Action Port : ActionPort  ActionPortLabel=if(u1 > u2)
  Out1 : Outport
  wires:
  In1/1 -> Out1/1

== system V2GStronge2_published_controller/Condition checker 4/If Action Subsystem33/If Action Subsystem1 ==
  In1 : Inport
  Action Port : ActionPort  ActionPortLabel=elseif( u1 < u2&u3>60)
  Out1 : Outport
  wires:
  In1/1 -> Out1/1

== system V2GStronge2_published_controller/Condition checker 4/If Action Subsystem33/If Action Subsystem2 ==
  In1 : Inport
  Action Port : ActionPort  ActionPortLabel=elseif(u1 < u2& u3<60)
  Out1 : Outport
  wires:
  In1/1 -> Out1/1
